simulink model "back_stoch_4dof"  (Simulink 8.5)
settings: Solver=ode3  StartTime=0.0  StopTime=10  RelTol=1e-3
undefined symbols (not defined in the file or in its folder): sample_time
settings Model: Creator=paulghanem  LastModifiedBy=User  CovSFcnEnable=off
settings DataIOCC: SignalLoggingSaveFormat=Dataset
settings OptimizationCC: ExpressionDepthLimit=128
settings DebuggingCC: UnderspecifiedInitializationDetection=Simplified  MergeDetectMultiDrivingBlocksExec=error  SolverPrmCheckMsg=warning  FcnCallInpInsideContextMsg=EnableAllAsError  StateNameClashWarn=none
settings GRTTargetCC: CombineOutputUpdateFcns=on  GRTInterface=off

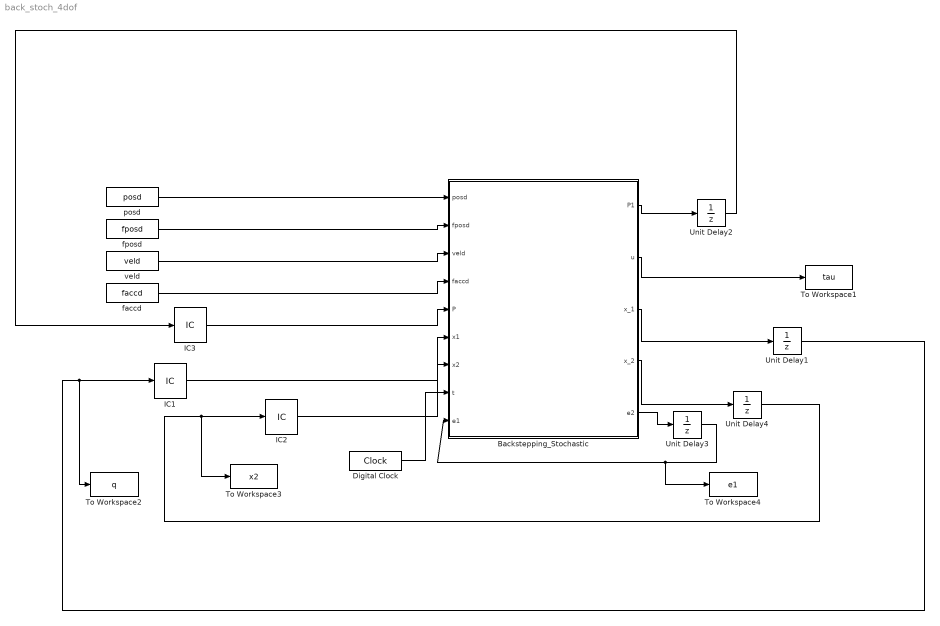
== system back_stoch_4dof ==
  Backstepping_Stochastic : MATLAB Function  TreatAsAtomicUnit=on
  Digital Clock : DigitalClock  SampleTime=sample_time
  IC1 : InitialCondition  Value=[0 -1.9 -0.1 3 ]
  IC2 : InitialCondition  Value=[0 0 0 0 ]
  IC3 : InitialCondition  Value=diag([1e-8 1e-10 1e-5 1e-9 1e-10 1e-10 1e-10 1e-10])
  To Workspace1 : ToWorkspace  VariableName=tau  SaveFormat=Structure With Time  SampleTime=-1
  To Workspace2 : ToWorkspace  VariableName=q  SaveFormat=Structure With Time  SampleTime=-1
  To Workspace3 : ToWorkspace  VariableName=x2  SaveFormat=Structure With Time  SampleTime=-1
  To Workspace4 : ToWorkspace  VariableName=e1  SaveFormat=Structure With Time  SampleTime=-1
  Unit Delay1 : UnitDelay  SampleTime=sample_time
  Unit Delay2 : UnitDelay  SampleTime=sample_time
  Unit Delay3 : UnitDelay  InitialCondition=[0 0 0 0 ]  SampleTime=sample_time
  Unit Delay4 : UnitDelay  SampleTime=sample_time
  faccd : FromWorkspace  VariableName=faccd  SampleTime=sample_time
  "fposd " : FromWorkspace  VariableName=fposd  SampleTime=sample_time
  "posd " : FromWorkspace  VariableName=posd  SampleTime=sample_time
  veld : FromWorkspace  VariableName=veld  SampleTime=sample_time
  wires:
  IC1/1 -> Backstepping_Stochastic/6(x1)
  IC2/1 -> Backstepping_Stochastic/7(x2)
  Backstepping_Stochastic/3(x_1) -> Unit Delay1/1
  Backstepping_Stochastic/4(x_2) -> Unit Delay4/1
  "posd "/1 -> Backstepping_Stochastic/1(posd)
  veld/1 -> Backstepping_Stochastic/3(veld)
  "fposd "/1 -> Backstepping_Stochastic/2(fposd)
  faccd/1 -> Backstepping_Stochastic/4(faccd)
  Backstepping_Stochastic/2(u) -> To Workspace1/1
  Unit Delay4/1 -> To Workspace3/1, IC2/1
  Unit Delay1/1 -> To Workspace2/1, IC1/1
  IC3/1 -> Backstepping_Stochastic/5(P)
  Backstepping_Stochastic/1(P1) -> Unit Delay2/1
  Unit Delay2/1 -> IC3/1
  Digital Clock/1 -> Backstepping_Stochastic/8(t)
  Backstepping_Stochastic/5(e2) -> Unit Delay3/1
  Unit Delay3/1 -> To Workspace4/1, Backstepping_Stochastic/9(e1)

== matlab function Backstepping_Stochastic ==
  data: P1 output double; posd input double; fposd input double; veld input double; faccd input double; P input double; u output double; x1 input double; x2 input double; x_1 output double; x_2 output double; t input double; e1 input double; e2 output double
function [P1,u,x_1,x_2,e2] = fcn(posd,fposd,veld,faccd,P,x1,x2,t,e1)
%#codegen
Ts=1/500;
sig = 2e-4;
R = 1e-12*eye(4);
Rp = 1e-3*eye(4);
q1 = 1*eye(4);
q2 = 1e-2*eye(4);
Q = 0*[q1 zeros(4);zeros(4) q2];
H = [eye(4) Ts*eye(4);zeros(4) eye(4)];
I1 = [zeros(4);eye(4)];
I2 = [eye(4);zeros(4)];
F1 =  diag([0.20519,0.094428,0.094428,0.03]);

   
 
 x11 = x1 + sig*(0.5 - rand(4,1));
 if t < 1
 e1=posd-x1;
 end
 e2=e1;
 
 posd=posd-e1;
 fposd=fposd-e1;
 
 
 
 
E = posd - x11;
Ed = fposd - x11;

K = Ts*I1'*P*inv(Ts^2*P + I1*Rp*I1' + (Ts*I2-I1)*R*(Ts*I2-I1)');
    K1 = 1*K(:,1:4);
    K2 = K(:,5:8);

 xx2=veld;
    Q22 = diag(diag(bq1(xx2)*bq1(xx2)'));
    Q = [zeros(4) zeros(4);zeros(4) Q22];
    PHI = H - Ts*I1*K;
    P1 = PHI*P*PHI' + I1*K*I1*Rp*I1'*K'*I1' + I1*K*(Ts*I2-I1)*R*(Ts*I2-I1)'*K'*I1' + Ts^2*I1*R*I1' + Ts^2*Q;
   
    
    x11=transpose(x11);
    ff = G1(x11);   
    
     u= ff + (D1(x11)+F1)*(faccd + K1*E + K2*(Ed - E)/Ts);
    
    %not to be used in real time
    U=u;
    
    x_1 =  x2*Ts + x1;
    x_2 = (-inv(D1(x1)+F1)*(G1(x1) + bq1(x2)) + inv(D1(x1)+F1)*U)*Ts + x2;
     
    
end 
function G1=G1(q)


DH_a = [0 0 0.045 -0.045];
    DH_d = [0 0 .55 0 ];
    DH_alpha = [-pi/2 pi/2 -pi/2 pi/2];

    m = [10.7676 3.87 1.8022 2.4];    
     
    com= zeros(3,4);
    
   com(:,1) = [-0.00443422;0.12189039;-0.00066489];
    com(:,2) = [-0.00236983;0.03105614;0.01542114 ];
    com(:,3) = [-0.03825858;0.20750770;0.00003309];
    com(:,4) = [0.00498512;-0.00022942;0.13271662 ];
 
        
     I=zeros(3,3,4);
    T=zeros(4,4,4);
     I(:,:,1) = [0.29486350,-0.00795023,-0.00009311;
                 -0.00795023,0.11350017,-0.00018711;
                -0.00009311,-0.00018711,0.25065343];
    I(:,:,2) =[0.02606840,-0.00001346,-0.00011701;
               -0.00001346,0.01472202,0.00003659;
              -0.00011701,0.00003659,0.01934814];
    I(:,:,3) = [0.13671601,-0.01680434, 0.00000510;
               -0.01680434,0.00588354,-0.00000530;
                0.00000510,-0.00000530,0.13951371];
    I(:,:,4) = [ 0.05719268,0.00001467,0.00008193;
                 0.00001467,0.05716470,-0.00009417;
                 0.00008193,-0.00009417,0.00300441] ;
    
            
             
             
for j=1:4,
        a = DH_a(j);
        d = DH_d(j);
        alpha = DH_alpha(j);
        T(:,:,j) = getTransformDH(a, d, alpha, q(j));
end 

comstar=zeros(4,4);

   
    comstar(:,1) = [com(:,1);1];
    comstar(:,2) = [com(:,2);1];
    comstar(:,3) = [com(:,3);1];
    comstar(:,4) = [com(:,4);1];
    
    Q=zeros(4,4);
    
    Q=[0,-1,0,0;
     1,0,0,0;
     0,0,0,0;
     0,0,0,0];
   
   
 gravity=[0,0,-9.81,0];
 G1=zeros(4,1);
   G1(1)= -m(1)*gravity*Q*T(:,:,1)*comstar(:,1)-m(2)*gravity*Q*T(:,:,1)*T(:,:,2)*comstar(:,2)-m(3)*gravity*Q*T(:,:,1)*T(:,:,2)*T(:,:,3)*comstar(:,3)-m(4)*gravity*Q*T(:,:,1)*T(:,:,2)*T(:,:,3)*T(:,:,4)*comstar(:,4);   
   G1(2)= -m(2)*gravity*T(:,:,1)*Q*T(:,:,2)*comstar(:,2)-m(3)*gravity*T(:,:,1)*Q*T(:,:,2)*T(:,:,3)*comstar(:,3)-m(4)*gravity*T(:,:,1)*Q*T(:,:,2)*T(:,:,3)*T(:,:,4)*comstar(:,4);
   G1(3)= -m(3)*gravity*T(:,:,1)*T(:,:,2)*Q*T(:,:,3)*comstar(:,3)-m(4)*gravity*T(:,:,1)*T(:,:,2)*Q*T(:,:,3)*T(:,:,4)*comstar(:,4);
   G1(4)= -m(4)*gravity*T(:,:,1)*T(:,:,2)*T(:,:,3)*Q*T(:,:,4)*comstar(:,4);
end 
    function T = getTransformDH(a,d,alpha,q)
    ct = cos(q);
    st = sin(q);
    cb = cos(alpha);
    sb = sin(alpha);
    
    T = [ ct, -st*cb,  st*sb, a*ct;
          st,  ct*cb, -ct*sb, a*st;
          0, sb, cb, d;
          0, 0, 0, 1 ];            
 end       
function bq1 = bq1(qd)



s=20;
bc = [2.516; 2.581; 2.038; 0.956];
B =  [1.142; 0.946; 0.309; 0.255];

bq1 = bc.*atan(s*qd)*2/pi+B.*qd;
end 

function D1 =D1(q);
DH_a = [0 0 0.045 -0.045];
    DH_d = [0 0 .55 0 ];
    DH_alpha = [-pi/2 pi/2 -pi/2 pi/2];

    m = [10.7676 3.87 1.8022 2.4];
    
     
    com= zeros(3,4);
    
   com(:,1) = [-0.00443422;0.12189039;-0.00066489];
    com(:,2) = [-0.00236983;0.03105614;0.01542114 ];
    com(:,3) = [-0.03825858;0.20750770;0.00003309];
    com(:,4) = [0.00498512;-0.00022942;0.13271662 ];
 
     
       
        
    I=zeros(3,3,4);
    T=zeros(4,4,4);
     I(:,:,1) = [0.29486350,-0.00795023,-0.00009311;
                 -0.00795023,0.11350017,-0.00018711;
                -0.00009311,-0.00018711,0.25065343];
    I(:,:,2) =[0.02606840,-0.00001346,-0.00011701;
               -0.00001346,0.01472202,0.00003659;
              -0.00011701,0.00003659,0.01934814];
    I(:,:,3) = [0.13671601,-0.01680434, 0.00000510;
               -0.01680434,0.00588354,-0.00000530;
                0.00000510,-0.00000530,0.13951371];
    I(:,:,4) = [ 0.05719268,0.00001467,0.00008193;
                 0.00001467,0.05716470,-0.00009417;
                 0.00008193,-0.00009417,0.00300441] ;
    
            
             
             
for j=1:4,
        a = DH_a(j);
        d = DH_d(j);
        alpha = DH_alpha(j);
        T(:,:,j) = getTransformDH(a, d, alpha, q(j));
end 

comstar=zeros(4,4);

   
    comstar(:,1) = [com(:,1);1];
    comstar(:,2) = [com(:,2);1];
    comstar(:,3) = [com(:,3);1];
    comstar(:,4) = [com(:,4);1];
    
    
    Q=zeros(4,4);
    
    Q=[0,-1,0,0;
     1,0,0,0;
     0,0,0,0;
     0,0,0,0];
   

   
U=zeros(4,4,4,4);
   
   U(:,:,1,1)= Q*T(:,:,1);
   U(:,:,2,1)= Q*T(:,:,1)*T(:,:,2);
   U(:,:,3,1)= Q*T(:,:,1)*T(:,:,2)*T(:,:,3);
   U(:,:,4,1)= Q*T(:,:,1)*T(:,:,2)*T(:,:,3)*T(:,:,4);
   
   
   U(:,:,2,2)= T(:,:,1)*Q*T(:,:,2);
   U(:,:,3,2)= T(:,:,1)*Q*T(:,:,2)*T(:,:,3);
   U(:,:,4,2)= T(:,:,1)*Q*T(:,:,2)*T(:,:,3)*T(:,:,4);
   
   
  
   U(:,:,3,3)= T(:,:,1)*T(:,:,2)*Q*T(:,:,3);
   U(:,:,4,3)= T(:,:,1)*T(:,:,2)*Q*T(:,:,3)*T(:,:,4);
   
   
   U(:,:,4,4)= T(:,:,1)*T(:,:,2)*T(:,:,3)*Q*T(:,:,4);
  
   
  
   
   
   
  
   J=zeros(4,4,4);
 
   
   J(:,:,1)=[0.5*(-I(1,1,1)+I(2,2,1)+I(3,3,1)), I(1,2,1), I(1,3,1), m(1)*com(1,1);
             I(1,2,1) ,0.5*(I(1,1,1)-I(2,2,1)+I(3,3,1)), I(2,3,1), m(1)*com(2,1);
             I(1,3,1), I(2,3,1), 0.5*(I(1,1,1)+I(2,2,1)-I(3,3,1)), m(1)*com(3,1);
              m(1)*com(1,1), m(1)*com(2,1), m(1)*com(3,1), m(1)];
   
    J(:,:,2)=[0.5*(-I(1,1,2)+I(2,2,2)+I(3,3,2)), I(1,2,2), I(1,3,2), m(2)*com(1,2);
             I(1,2,2) ,0.5*(I(1,1,2)-I(2,2,2)+I(3,3,2)), I(2,3,2), m(2)*com(2,2);
             I(1,3,2), I(2,3,2), 0.5*(I(1,1,2)+I(2,2,2)-I(3,3,2)), m(2)*com(3,2);
              m(2)*com(1,2), m(2)*com(2,2), m(2)*com(3,2), m(2)];
   
          
     J(:,:,3)=[0.5*(-I(1,1,3)+I(2,2,3)+I(3,3,3)), I(1,2,3), I(1,3,3), m(3)*com(1,3);
             I(1,2,3) ,0.5*(I(1,1,3)-I(2,2,3)+I(3,3,3)), I(2,3,3), m(3)*com(2,3);
             I(1,3,3), I(2,3,3), 0.5*(I(1,1,3)+I(2,2,3)-I(3,3,3)), m(3)*com(3,3);
              m(3)*com(1,3), m(3)*com(2,3), m(3)*com(3,3), m(3)];      
   
   
    J(:,:,4)=[0.5*(-I(1,1,4)+I(2,2,4)+I(3,3,4)), I(1,2,4), I(1,3,4), m(4)*com(1,4);
             I(1,2,4) ,0.5*(I(1,1,4)-I(2,2,4)+I(3,3,4)), I(2,3,4), m(4)*com(2,4);
             I(1,3,4), I(2,3,4), 0.5*(I(1,1,4)+I(2,2,4)-I(3,3,4)), m(4)*com(3,4);
              m(4)*com(1,4), m(4)*com(2,4), m(4)*com(3,4), m(4)];
   
   
   
          
          D1=zeros(4,4);
   
   
    D1(1,1)= trace(U(:,:,1,1)*J(:,:,1)*transpose(U(:,:,1,1))) + trace(U(:,:,2,1)*J(:,:,2)*transpose(U(:,:,2,1))) + trace(U(:,:,3,1)*J(:,:,3)*transpose(U(:,:,3,1))) + trace(U(:,:,4,1)*J(:,:,4)*transpose(U(:,:,4,1))) ;
    D1(1,2)= trace(U(:,:,2,2)*J(:,:,2)*transpose(U(:,:,2,1))) + trace(U(:,:,3,2)*J(:,:,3)*transpose(U(:,:,3,1))) + trace(U(:,:,4,2)*J(:,:,4)*transpose(U(:,:,4,1))) ; 
    D1(1,3)= trace(U(:,:,3,3)*J(:,:,3)*transpose(U(:,:,3,1)))+ trace(U(:,:,4,3)*J(:,:,4)*transpose(U(:,:,4,1))); 
    D1(1,4)= trace(U(:,:,4,4)*J(:,:,4)*transpose(U(:,:,4,1)));
    
    
    D1(2,1)= trace(U(:,:,2,1)*J(:,:,2)*transpose(U(:,:,2,2)))+ trace(U(:,:,3,1)*J(:,:,3)*transpose(U(:,:,3,2)))+ trace(U(:,:,4,1)*J(:,:,4)*transpose(U(:,:,4,2)));
    D1(2,2)= trace(U(:,:,2,2)*J(:,:,2)*transpose(U(:,:,2,2)))+ trace(U(:,:,3,2)*J(:,:,3)*transpose(U(:,:,3,2)))+ trace(U(:,:,4,2)*J(:,:,4)*transpose(U(:,:,4,2)));
    D1(2,3)= trace(U(:,:,3,3)*J(:,:,3)*transpose(U(:,:,3,2)))+ trace(U(:,:,4,3)*J(:,:,4)*transpose(U(:,:,4,2))); 
    D1(2,4)= trace(U(:,:,4,4)*J(:,:,4)*transpose(U(:,:,4,2))); 
    
    D1(3,1)= trace(U(:,:,3,1)*J(:,:,3)*transpose(U(:,:,3,3)))+ trace(U(:,:,4,1)*J(:,:,4)*transpose(U(:,:,4,3)));
    D1(3,2)= trace(U(:,:,3,2)*J(:,:,3)*transpose(U(:,:,3,3)))+ trace(U(:,:,4,2)*J(:,:,4)*transpose(U(:,:,4,3)));
    D1(3,3)= trace(U(:,:,3,3)*J(:,:,3)*transpose(U(:,:,3,3)))+ trace(U(:,:,4,3)*J(:,:,4)*transpose(U(:,:,4,3)));
    D1(3,4)= trace(U(:,:,4,4)*J(:,:,4)*transpose(U(:,:,4,3)));
    
     
     
    D1(4,1)= trace(U(:,:,4,1)*J(:,:,4)*transpose(U(:,:,4,4))); 
    D1(4,2)= trace(U(:,:,4,2)*J(:,:,4)*transpose(U(:,:,4,4))); 
    D1(4,3)= trace(U(:,:,4,3)*J(:,:,4)*transpose(U(:,:,4,4)));
    D1(4,4)= trace(U(:,:,4,4)*J(:,:,4)*transpose(U(:,:,4,4)));
    
end
